simulink model "airspeed_from_throttle"  (R2019a)
settings: Solver=VariableStepAuto  StartTime=0.0  StopTime=1000  RelTol=1e-3
values from neighbouring files (symbols this model uses):
  trans_func = [T_phi_delta_a T_chi_phi T_theta_delta_e T_h_theta T_h_Va T_Va_delta_t T_Va_theta T_v_delta_r]    [vtol_parameters.m]    (also in vtol_parameters_1.m)
undefined symbols (not defined in the file or in its folder): AP
settings Model: Creator=nikhil  LastModifiedBy=VTOL_HYD

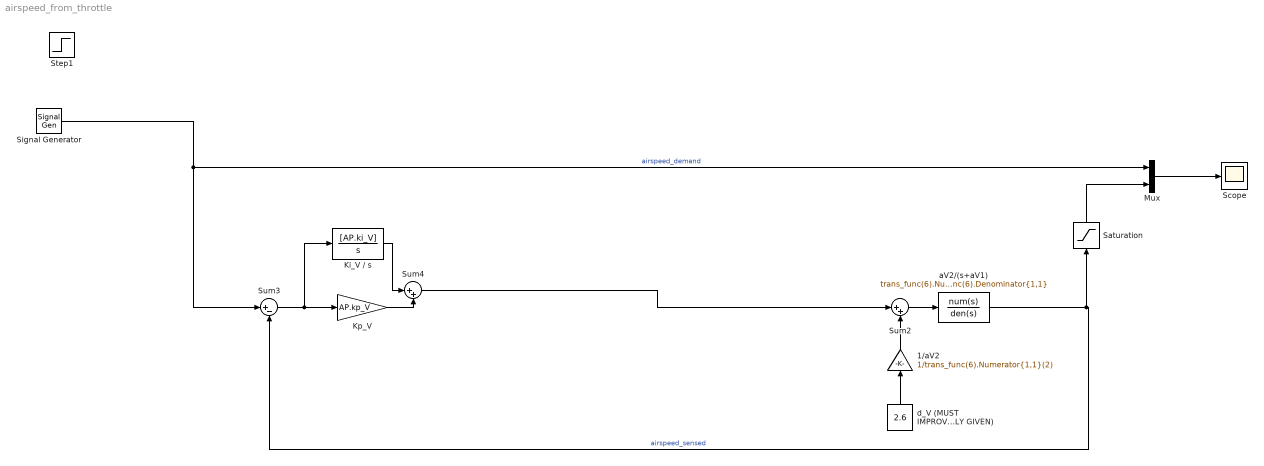
== system airspeed_from_throttle ==
  1/aV2 : Gain  Gain=1/trans_func(6).Numerator{1,1}(2)
  Ki_V / s : TransferFcn  Numerator=[AP.ki_V]  Denominator=[1 0]
  Kp_V : Gain  Gain=AP.kp_V
  Mux : Mux  Inputs=2
  Saturation : Saturate  UpperLimit=200  LowerLimit=-200
  Scope : Scope
  Signal Generator : SignalGenerator  WaveForm=square  Amplitude=35  Frequency=.08  Units=rad/sec
  Step1 : Step  Time=8  After=35  SampleTime=8
  Sum2 : Sum  Inputs=|++
  Sum3 : Sum  Inputs=|+-
  Sum4 : Sum  Inputs=|++
  aV2/(s+aV1) : TransferFcn  Numerator=trans_func(6).Numerator{1,1}(2)  Denominator=trans_func(6).Denominator{1,1}
  d_V (MUST IMPROVE! FORMULA NOT FULLY GIVEN) : Constant  Value=2.6
  wires:
  aV2/(s+aV1)/1 -> Saturation/1, Sum3/2  "airspeed_sensed"
  Mux/1 -> Scope/1
  Sum4/1 -> Sum2/1
  Ki_V / s/1 -> Sum4/1
  Kp_V/1 -> Sum4/2
  Signal Generator/1 -> Sum3/1, Mux/1  "airspeed_demand"
  Sum3/1 -> Ki_V / s/1, Kp_V/1
  1/aV2/1 -> Sum2/2
  d_V (MUST IMPROVE! FORMULA NOT FULLY GIVEN)/1 -> 1/aV2/1
  Sum2/1 -> aV2/(s+aV1)/1
  Saturation/1 -> Mux/2
